simulink model "P5_Modelo_ContrIntDiscret"  (R2025b)
settings: Solver=ode45  StartTime=0.0  StopTime=2  MaxStep=0.0001  RelTol=1e-3
undefined symbols (not defined in the file): C, f, F, G, Kdis, ke, Kidis, Ldis, p, theta0, thetaref, w0
settings Model: Creator=lucas

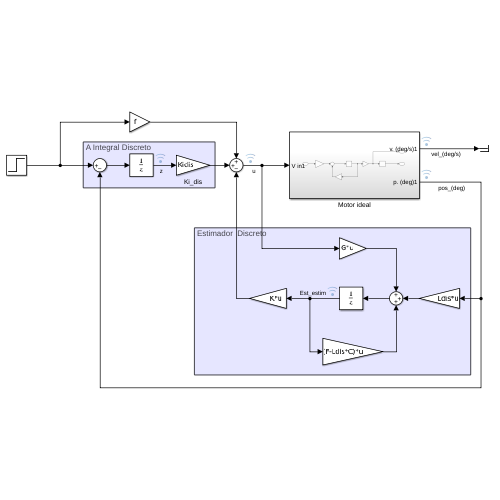
[thumbnail: Simulink's stored preview of the top-level diagram]
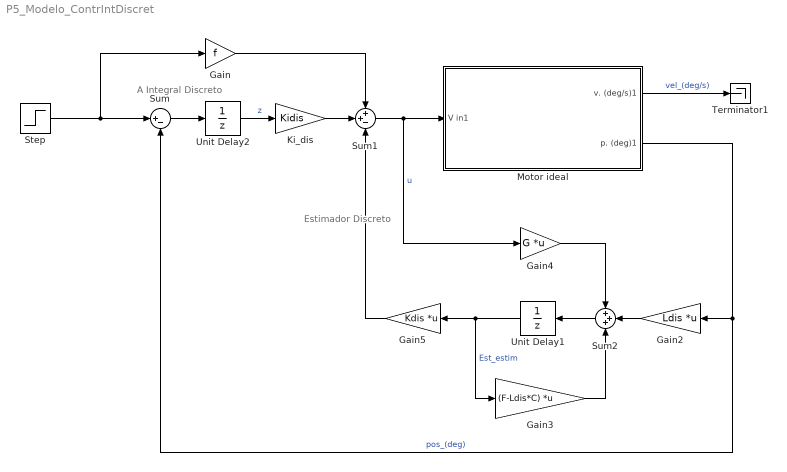
== system P5_Modelo_ContrIntDiscret ==
  note: A Integral Discreto
  note: Estimador Discreto
  Gain : Gain  Gain=f
  Gain2 : Gain  Gain=Ldis  Multiplication=Matrix(K*u)
  Gain3 : Gain  Gain=(F-Ldis*C)  Multiplication=Matrix(K*u)
  Gain4 : Gain  Gain=G  Multiplication=Matrix(K*u)
  Gain5 : Gain  Gain=Kdis  Multiplication=Matrix(K*u)
  Ki_dis : Gain  Gain=Kidis
  Motor ideal : Subsystem
  Step : Step  Time=0  Before=thetaref  After=thetaref  SampleTime=0
  Sum : Sum  Inputs=|+-
  Sum1 : Sum  Inputs=++-
  Sum2 : Sum  Inputs=+++
  Terminator1 : Terminator
  Unit Delay1 : UnitDelay  SampleTime=0.0001  HasFrameUpgradeWarning=on
  Unit Delay2 : UnitDelay  SampleTime=0.0001  HasFrameUpgradeWarning=on
  wires:
  Step/1 -> Sum/1, Gain/1
  Sum/1 -> Unit Delay2/1
  Unit Delay2/1 -> Ki_dis/1  "z"
  Gain/1 -> Sum1/1
  Ki_dis/1 -> Sum1/2
  Sum1/1 -> Gain4/1, Motor ideal/1(V in1)  "u"
  Gain4/1 -> Sum2/1
  Gain2/1 -> Sum2/2
  Sum2/1 -> Unit Delay1/1
  Gain3/1 -> Sum2/3
  Unit Delay1/1 -> Gain5/1, Gain3/1  "Est_estim"
  Gain5/1 -> Sum1/3
  Motor ideal/1(v. (deg/s)1) -> Terminator1/1  "vel_(deg/s)"
  Motor ideal/2(p. (deg)1) -> Gain2/1, Sum/2  "pos_(deg)"

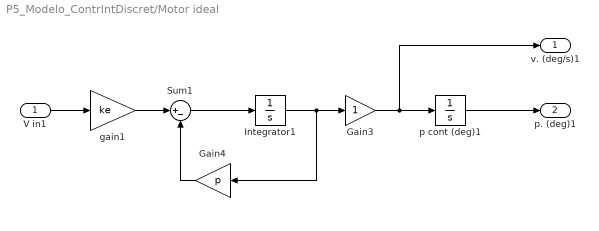
== system P5_Modelo_ContrIntDiscret/Motor ideal ==
  V in1 : Inport
  Gain3 : Gain
  Gain4 : Gain  Gain=p
  Integrator1 : Integrator  InitialCondition=w0
  Sum1 : Sum  Inputs=|+-
  gain1 : Gain  Gain=ke
  p cont (deg)1 : Integrator  InitialCondition=theta0
  v. (deg/s)1 : Outport
  p. (deg)1 : Outport  Port=2
  wires:
  Integrator1/1 -> Gain4/1, Gain3/1
  Sum1/1 -> Integrator1/1
  p cont (deg)1/1 -> p. (deg)1/1
  Gain3/1 -> v. (deg/s)1/1, p cont (deg)1/1
  V in1/1 -> gain1/1
  Gain4/1 -> Sum1/2
  gain1/1 -> Sum1/1
